simulink model "TransitiontoMultipleDestinations_2018a"  (R2018a)
settings: Solver=VariableStepAuto  StartTime=0.0  StopTime=10.0  RelTol=1e-3
settings Model: Creator=apple  LastModifiedBy=apple
settings DataIOCC: ReturnWorkspaceOutputs=on
settings SFSimCC: SimUseLocalCustomCode=on
settings RTWCC: RTWUseLocalCustomCode=on

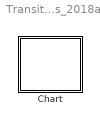
== system TransitiontoMultipleDestinations_2018a ==
  Chart : Stateflow chart  TreatAsAtomicUnit=on

== stateflow chart TransitiontoMultipleDestinations_2018a/Chart ==
  state B
    en:fprintf("Entry B");
    du:fprintf("During B");
    ex:fprintf("Exit B");
  state A
    en:fprintf("Entry A");
    du:fprintf("During A");
    ex:fprintf("Exit A");
  state C
    en:fprintf("Entry C");
    du:fprintf("During C");
    ex:fprintf("Exit A");
  (default) -> A
  (junction 3) -> B [order 1] : E_one
  A -> (junction 3)
  (junction 3) -> C [order 2] : E_two
  events: E_one local FUNCTION_CALL_EVENT; E_two local FUNCTION_CALL_EVENT
